simulink model "inch"  (R2023b)
settings: Solver=FixedStepAuto  StartTime=0.0  StopTime=30  RelTol=1e-3
model workspace: external: MAT-File C:\Users\Master\Desktop\seoultech_MRL\Impedance_inchworm\model_analysis\inch.mat (data not in the file)
values from neighbouring files (symbols this model uses):
  admit_d_x = 1    [inch.m]
  admit_d_z = 1    [inch.m]
  admit_k_x = 1    [inch.m]
  admit_k_z = 1    [inch.m]
  admit_m_x = 1    [inch.m]
  admit_m_z = 1    [inch.m]
  CoM1 = 0.13475    [inch.m]
  CoM2 = 0.0562    [inch.m]
  g = 9.80665    [inch.m]
  K_sp1 = 11.8    [inch.m]
  K_sp2 = 5.7    [inch.m]
  L1 = 0.24215    [inch.m]
  L2 = 0.1759    [inch.m]
  m1 = 0.420    (= 0.42)    [inch.m]
  m2 = 0.225    [inch.m]
  w_c = 30    [inch.m]
settings Model: Creator=seosu  LastModifiedBy=Master
settings RTWCC: GPUComputeCapability=5.0

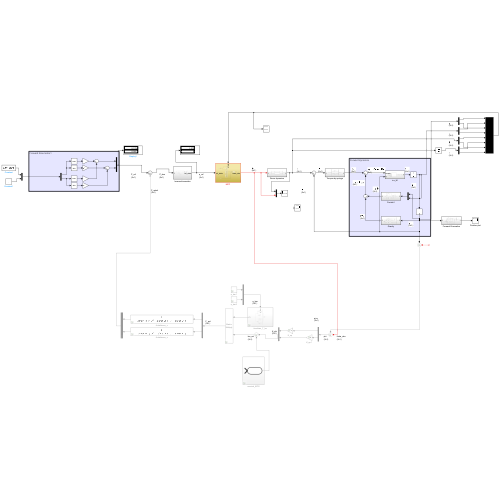
[thumbnail: Simulink's stored preview of the top-level diagram]
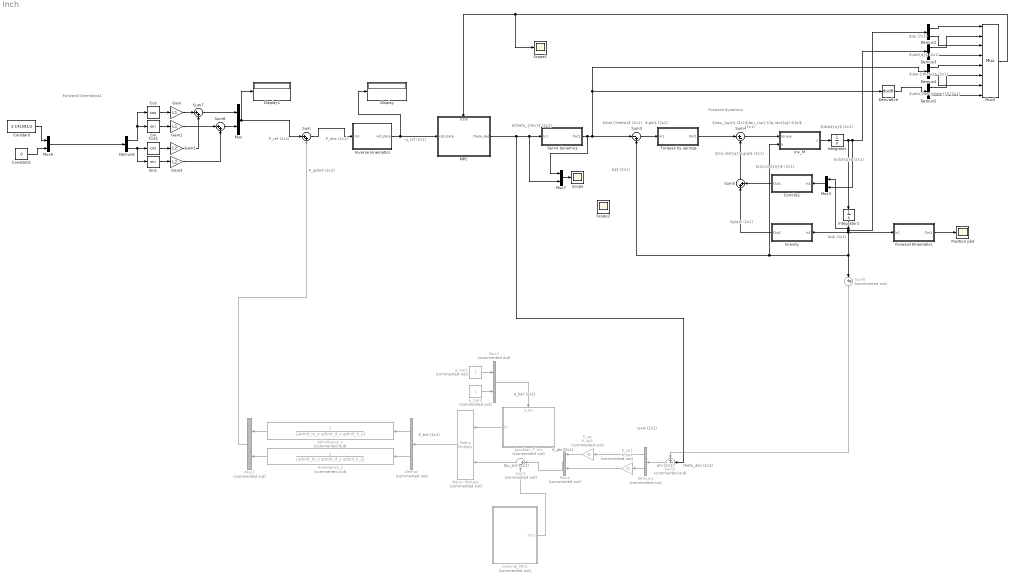
== system inch ==
  note: Forward Kinematics1
  note: P_ref
      | (2x1)
  note: q+w
      | (2x1)
  note: theta_des
      | (2x1)
  note: phi
      | (2x1)
  note: K_phi
      | (2x1)
  note: tau_ext
      | (2x1)
  note: F_ext
      | (2x1)
  note: q_bar
      | (2x1)
  note: P_admit
      | (2x1)
  note: P_des
      | (2x1)
  note: Forward dynamics
  note: q_ref
      | (2x1)
  note: $\theta_{des}$
      | (2x1)
  note: $\bar{\theta}$
      | (2x1)
  note: $q$
      | (2x1)
  note: $\phi$
      | (2x1)
  note: $\tau_{sp}$
      | (2x1)
  note: $\tau_{sp}-C(q,\dot{q})-G(q)$
      | (2x1)
  note: $g(q)$
      | (2x1)
  note: $c(q,\dot{q})$
      | (2x1)
  note: $c(q,\dot{q})+g(q)$
      | (2x1)
  note: $\ddot{q}$
      | (2x1)
  note: $\dot{q}$
      | (2x1)
  note: $q$
      | (2x1)
  note: $q$
      | (2x1)
  note: $\dot{q}$
      | (2x1)
  note: $\bar{\theta}$
      | (2x1)
  note: $\dot{\bar{\theta}}$
      | (2x1)
  Admittance_x : TransferFcn  Commented=on  Denominator=[admit_m_x admit_d_x admit_k_x]
  Admittance_z : TransferFcn  Commented=on  Denominator=[admit_m_z admit_d_z admit_k_z]
  Constant : Constant  Value=3.141592/2
  Constant1 : Constant  Value=0
  Coriolis1 : Subsystem
  Cos : Trigonometry  Operator=cos
  Cos1 : Trigonometry  Operator=cos
  Demux : Demux  Commented=on  Outputs=2
  Demux1 : Demux  Commented=on  Outputs=2
  Demux{2..6} (5 alike) : Demux  Outputs=2
  Derivative : Derivative
  Display : Display
  Display1 : Display
  Forward Kinematics : Subsystem
  Gain : Gain  Gain=L1
  Gain1 : Gain  Gain=L1
  Gain2 : Gain  Gain=L2
  Gain3 : Gain  Gain=L2
  Gravity : Subsystem
  Integrator : Integrator
  Integrator1 : Integrator
  Inverse kinematics : Subsystem
  Jacobian_T_Inv : Subsystem  Commented=on
      settings: PortSchema="{\"entries\":[{\"content\":{\"sides\":[{\"content\":{},\"type\":\"ConnectorPlacement.EquallySpacedRectSide\",\"uuid\":\"e35815a1-46bf-4be5-848e-f0ce23dcfc5f\"},{\"content\":{\"connectorIds\":[\"Out1\"],\"side\":\"RIGHT\"},\"type\":\"ConnectorPlacement.EquallySpacedRectSide\",\"uuid\":\"475e0ecd-9b25-4f4d-9a47-e60ebdf6c1c0\"},{\"content\":{\"connectorIds\":[\"In1\"],\"side\":\"TOP\"},\"type\":\"ConnectorPlacement.EquallySpacedRectSide\",\"uuid\":\"24b4edd2-9023-4e45-b53e-92ef1b268f51\"}]},\"type\":\"ConnectorPlacement.EquallySpacedConnector\",\"uuid\":\"0e42b979-70d4-4e07-81ad-a6fcf3fd88d3\"}],\"packageUris\":[\"http://schema.mathworks.com/mf0/Connector/R2020b\"],\"version\":\"1.0\"}"
  K_sp : Gain  Commented=on  Gain=K_sp1
  K_sp1 : Gain  Commented=on  Gain=K_sp2
  MPC : Subsystem
      settings: PortSchema="{\"entries\":[{\"content\":{\"sides\":[{\"content\":{\"connectorIds\":[\"In1\"]},\"type\":\"ConnectorPlacement.EquallySpacedRectSide\",\"uuid\":\"faaa2caa-5b70-4c85-ac0e-3ca1c201351b\"},{\"content\":{\"connectorIds\":[\"Out1\"],\"side\":\"RIGHT\"},\"type\":\"ConnectorPlacement.EquallySpacedRectSide\",\"uuid\":\"30f98641-3e3d-4ab7-bed4-d131e440aef7\"},{\"content\":{\"connectorIds\":[\"In2\"],\"side\":\"TOP\"},\"type\":\"ConnectorPlacement.EquallySpacedRectSide\",\"uuid\":\"cc9bccd0-31f7-44f6-a189-fb05f25d7f1a\"}]},\"type\":\"ConnectorPlacement.EquallySpacedConnector\",\"uuid\":\"92c981b0-7f9b-49a2-b6f3-a82ac2dd5f41\"}],\"packageUris\":[\"http://schema.mathworks.com/mf0/Connector/R2020b\"],\"version\":\"1.0\"}"
  Matrix Multiply : Product  Commented=on  Multiplication=Matrix(*)
  Mux{,3,6..7} (4 alike) : Mux  Inputs=2
  Mux1 : Mux  Commented=on  Inputs=2
  Mux2 : Mux  Commented=on  Inputs=2
  Mux4 : Mux  Commented=on  Inputs=2
  Mux5 : Mux  Inputs=8
  Position plot : Scope
  Scope : Scope
  Scope1 : Scope
  Scope2 : Scope
  Servo dynamics : Subsystem
  Sin : Trigonometry
  Sin1 : Trigonometry
  Sum{,5,7..8} (4 alike) : Sum  Inputs=|++
  Sum1 : Sum  Commented=on  Inputs=|+-
  Sum2 : Sum  Commented=on  Inputs=+-|
  Sum3 : Sum  Inputs=|-+
  Sum4 : Sum  Inputs=|+-
  Sum6 : Sum  Commented=on  Inputs=|++
  Torques by springs : Subsystem
  inv_M : Subsystem
  nominal_MCG : Subsystem  Commented=on
  q_bar1 : Constant  Commented=on  Value=2
  q_bar2 : Constant  Commented=on
  wires:
  Mux/1 -> Sum/1, Display1/1
  Mux2/1 -> Jacobian_T_Inv/1(q_bar)
  Jacobian_T_Inv/1(JTI) -> Matrix Multiply/1
  Matrix Multiply/1 -> Demux/1
  Sum1/1 -> Matrix Multiply/2
  nominal_MCG/1(Out1) -> Sum1/2
  Sum2/1 -> Demux1/1
  Integrator1/1 -> inv_M/2(q), Sum3/2, Sum6/1, Gravity/1(In1), Forward Kinematics/1(In1), Demux2/1, Mux3/1
  Admittance_x/1 -> Mux1/1
  Demux/2 -> Admittance_z/1
  Admittance_z/1 -> Mux1/2
  Demux/1 -> Admittance_x/1
  q_bar1/1 -> Mux2/1
  q_bar2/1 -> Mux2/2
  MPC/1(theta_des) -> Mux7/2, Servo dynamics/1(In1), Sum2/2
  Torques by springs/1(Out1) -> Sum4/1
  Sum4/1 -> inv_M/1(torque)
  Sum3/1 -> Torques by springs/1(In1)
  Derivative/1 -> Demux5/1
  inv_M/1(y) -> Integrator/1
  Integrator/1 -> Demux3/1, Mux3/2, Integrator1/1
  Forward Kinematics/1(Out1) -> Position plot/1
  Sum5/1 -> Sum4/2
  Servo dynamics/1(Out1) -> Mux7/1, Demux4/1, Derivative/1, Sum3/1
  Gravity/1(Out1) -> Sum5/1
  Coriolis1/1(Out1) -> Sum5/2
  Sum6/1 -> Sum2/1
  ? -> Sum6/2
  Mux3/1 -> Coriolis1/1(In1)
  Demux1/1 -> K_sp/1
  Demux1/2 -> K_sp1/1
  K_sp1/1 -> Mux4/2
  K_sp/1 -> Mux4/1
  Mux4/1 -> Sum1/1
  Inverse kinematics/1(ref_state) -> Display/1, MPC/1(ref_state)
  Sum/1 -> Inverse kinematics/1(In1)
  Demux2/1 -> Mux5/1
  Demux2/2 -> Mux5/3
  Demux3/1 -> Mux5/2
  Demux3/2 -> Mux5/4
  Demux4/1 -> Mux5/5
  Demux5/1 -> Mux5/6
  Demux4/2 -> Mux5/7
  Demux5/2 -> Mux5/8
  Mux5/1 -> Scope1/1, MPC/2(state)
  Sum8/1 -> Mux/2
  Sum7/1 -> Mux/1
  Gain3/1 -> Sum8/2
  Gain1/1 -> Sum8/1
  Gain/1 -> Sum7/1
  Gain2/1 -> Sum7/2
  Sin/1 -> Gain1/1
  Sin1/1 -> Gain3/1
  Cos1/1 -> Gain2/1
  Cos/1 -> Gain/1
  Demux6/2 -> Sin1/1, Cos1/1
  Demux6/1 -> Cos/1, Sin/1
  Mux6/1 -> Demux6/1
  Constant/1 -> Mux6/1
  Constant1/1 -> Mux6/2
  Mux7/1 -> Scope/1
  Mux1/1 -> Sum/2

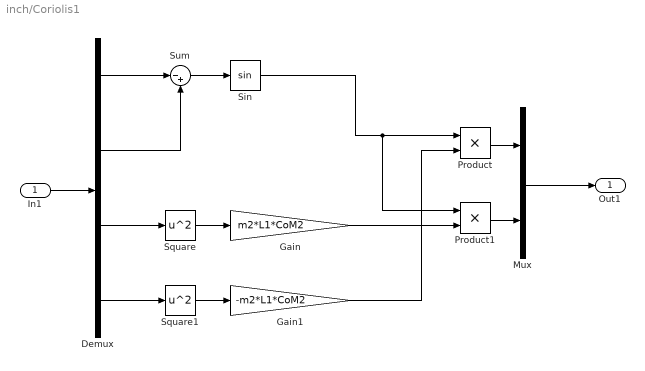
== system inch/Coriolis1 ==
  In1 : Inport
  Demux : Demux
  Gain : Gain  Gain=m2*L1*CoM2
  Gain1 : Gain  Gain=-m2*L1*CoM2
  Mux : Mux  Inputs=2
  Product : Product
  Product1 : Product
  Sin : Trigonometry
  Square : Math  Operator=square  SignedPower=on  RndMeth=Zero
  Square1 : Math  Operator=square  SignedPower=on  RndMeth=Zero
  Sum : Sum  Inputs=|-+
  Out1 : Outport
  wires:
  In1/1 -> Demux/1
  Demux/2 -> Sum/2
  Demux/1 -> Sum/1
  Sum/1 -> Sin/1
  Demux/3 -> Square/1
  Demux/4 -> Square1/1
  Square/1 -> Gain/1
  Square1/1 -> Gain1/1
  Sin/1 -> Product1/1, Product/1
  Gain/1 -> Product1/2
  Gain1/1 -> Product/2
  Product1/1 -> Mux/2
  Product/1 -> Mux/1
  Mux/1 -> Out1/1

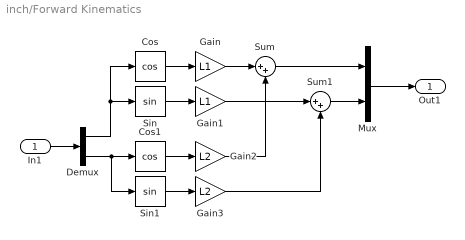
== system inch/Forward Kinematics ==
  In1 : Inport
  Cos : Trigonometry  Operator=cos
  Cos1 : Trigonometry  Operator=cos
  Demux : Demux  Outputs=2
  Gain : Gain  Gain=L1
  Gain1 : Gain  Gain=L1
  Gain2 : Gain  Gain=L2
  Gain3 : Gain  Gain=L2
  Mux : Mux  Inputs=2
  Sin : Trigonometry
  Sin1 : Trigonometry
  Sum : Sum  Inputs=|++
  Sum1 : Sum  Inputs=|++
  Out1 : Outport
  wires:
  In1/1 -> Demux/1
  Mux/1 -> Out1/1
  Demux/1 -> Cos/1, Sin/1
  Demux/2 -> Sin1/1, Cos1/1
  Cos/1 -> Gain/1
  Cos1/1 -> Gain2/1
  Sin1/1 -> Gain3/1
  Sin/1 -> Gain1/1
  Gain2/1 -> Sum/2
  Gain/1 -> Sum/1
  Gain1/1 -> Sum1/1
  Gain3/1 -> Sum1/2
  Sum/1 -> Mux/1
  Sum1/1 -> Mux/2

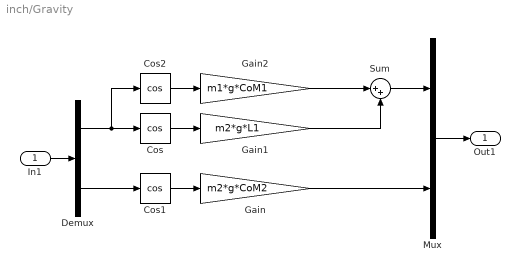
== system inch/Gravity ==
  In1 : Inport
  Cos : Trigonometry  Operator=cos
  Cos1 : Trigonometry  Operator=cos
  Cos2 : Trigonometry  Operator=cos
  Demux : Demux  Outputs=2
  Gain : Gain  Gain=m2*g*CoM2
  Gain1 : Gain  Gain=m2*g*L1
  Gain2 : Gain  Gain=m1*g*CoM1
  Mux : Mux  Inputs=2
  Sum : Sum  Inputs=|++
  Out1 : Outport
  wires:
  In1/1 -> Demux/1
  Demux/2 -> Cos1/1
  Cos1/1 -> Gain/1
  Cos2/1 -> Gain2/1
  Cos/1 -> Gain1/1
  Demux/1 -> Cos2/1, Cos/1
  Gain2/1 -> Sum/1
  Gain1/1 -> Sum/2
  Gain/1 -> Mux/2
  Sum/1 -> Mux/1
  Mux/1 -> Out1/1

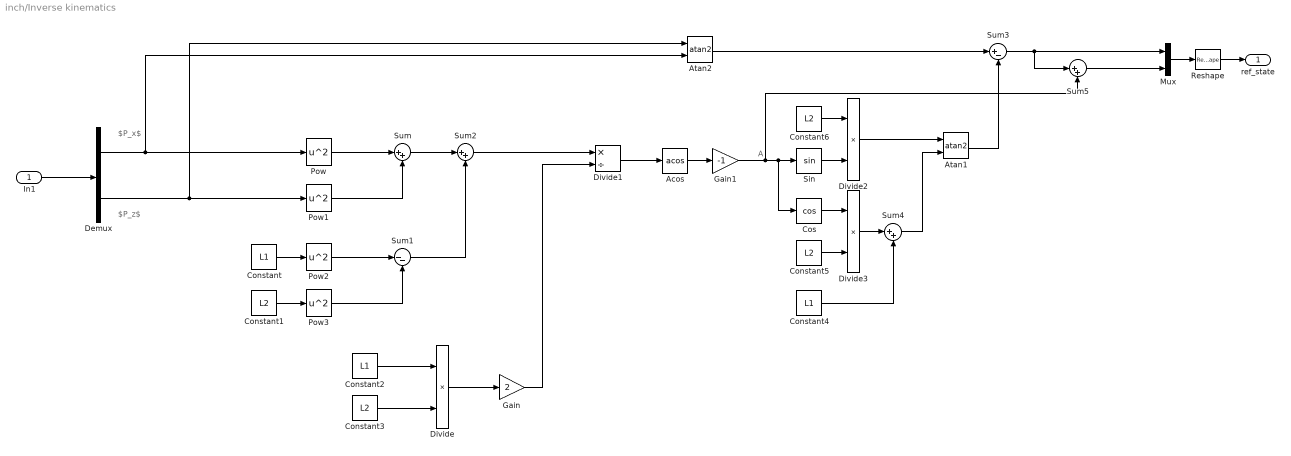
== system inch/Inverse kinematics ==
  note: A
  note: $P_x$
  note: $P_z$
  In1 : Inport
  Acos : Trigonometry  Operator=acos
  Atan1 : Trigonometry  Operator=atan2
  Atan2 : Trigonometry  Operator=atan2
  Constant : Constant  Value=L1
  Constant{1,3,5..6} (4 alike) : Constant  Value=L2
  Constant2 : Constant  Value=L1
  Constant4 : Constant  Value=L1
  Cos : Trigonometry  Operator=cos
  Demux : Demux  Outputs=2
  Divide : Product  Inputs=**
  Divide1 : Product  Inputs=*/
  Divide2 : Product  Inputs=**
  Divide3 : Product  Inputs=**
  Gain : Gain  Gain=2
  Gain1 : Gain  Gain=-1
  Mux : Mux  Inputs=2
  Pow{,1..3} (4 alike) : Math  Operator=square  SignedPower=on  RndMeth=Zero
  Reshape : Reshape  OutputDimensionality=Column vector (2-D)
  Sin : Trigonometry
  Sum{,2,4..5} (4 alike) : Sum  Inputs=|++
  Sum1 : Sum  Inputs=|--
  Sum3 : Sum  Inputs=|+-
  ref_state : Outport
  wires:
  In1/1 -> Demux/1
  Demux/1 -> Pow/1, Atan2/2
  Demux/2 -> Atan2/1, Pow1/1
  Pow/1 -> Sum/1
  Pow1/1 -> Sum/2
  Constant/1 -> Pow2/1
  Constant1/1 -> Pow3/1
  Pow2/1 -> Sum1/1
  Pow3/1 -> Sum1/2
  Sum/1 -> Sum2/1
  Sum1/1 -> Sum2/2
  Sum2/1 -> Divide1/1
  Constant2/1 -> Divide/1
  Constant3/1 -> Divide/2
  Divide/1 -> Gain/1
  Gain/1 -> Divide1/2
  Divide1/1 -> Acos/1
  Acos/1 -> Gain1/1
  Atan2/1 -> Sum3/1
  Gain1/1 -> Sum5/2, Cos/1, Sin/1
  Constant5/1 -> Divide3/2
  Cos/1 -> Divide3/1
  Divide3/1 -> Sum4/1
  Constant4/1 -> Sum4/2
  Sin/1 -> Divide2/2
  Constant6/1 -> Divide2/1
  Sum4/1 -> Atan1/2
  Divide2/1 -> Atan1/1
  Atan1/1 -> Sum3/2
  Sum3/1 -> Sum5/1, Mux/1
  Sum5/1 -> Mux/2
  Mux/1 -> Reshape/1
  Reshape/1 -> ref_state/1

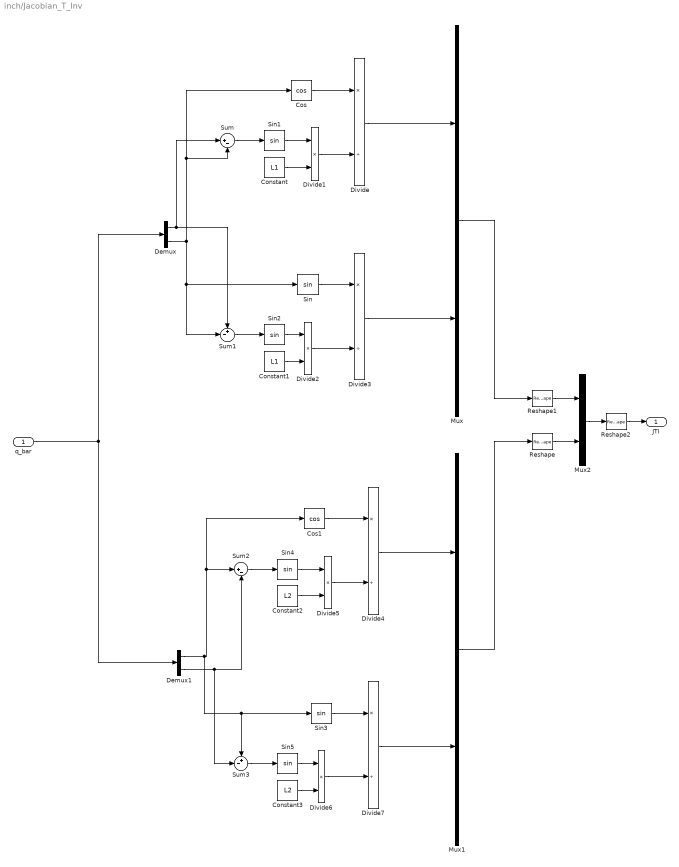
== system inch/Jacobian_T_Inv ==
  q_bar : Inport
  Constant : Constant  Value=L1
  Constant1 : Constant  Value=L1
  Constant2 : Constant  Value=L2
  Constant3 : Constant  Value=L2
  Cos : Trigonometry  Operator=cos
  Cos1 : Trigonometry  Operator=cos
  Demux : Demux  Outputs=2
  Demux1 : Demux  Outputs=2
  Divide{,3..4,7} (4 alike) : Product  Inputs=*/
  Divide{1..2,5..6} (4 alike) : Product  Inputs=**
  Mux : Mux  Inputs=2
  Mux1 : Mux  Inputs=2
  Mux2 : Mux  Inputs=2
  Reshape : Reshape  OutputDimensionality=Column vector (2-D)
  Reshape1 : Reshape  OutputDimensionality=Column vector (2-D)
  Reshape2 : Reshape  OutputDimensionality=Customize  OutputDimensions=[2,2]
  Sin{,1..5} (6 alike) : Trigonometry
  Sum : Sum  Inputs=|+-
  Sum1 : Sum  Inputs=+-|
  Sum2 : Sum  Inputs=|+-
  Sum3 : Sum  Inputs=+-|
  JTI : Outport
  wires:
  q_bar/1 -> Demux1/1, Demux/1
  Demux/2 -> Sum1/2, Sin/1, Sum/2, Cos/1
  Cos/1 -> Divide/1
  Demux/1 -> Sum/1, Sum1/1
  Sum/1 -> Sin1/1
  Sin1/1 -> Divide1/1
  Constant/1 -> Divide1/2
  Divide1/1 -> Divide/2
  Sum1/1 -> Sin2/1
  Constant1/1 -> Divide2/2
  Sin2/1 -> Divide2/1
  Divide2/1 -> Divide3/2
  Sin/1 -> Divide3/1
  Divide3/1 -> Mux/2
  Divide/1 -> Mux/1
  Divide7/1 -> Mux1/2
  Sin5/1 -> Divide6/1
  Sum3/1 -> Sin5/1
  Constant3/1 -> Divide6/2
  Divide4/1 -> Mux1/1
  Sin3/1 -> Divide7/1
  Divide6/1 -> Divide7/2
  Divide5/1 -> Divide4/2
  Sin4/1 -> Divide5/1
  Demux1/1 -> Sin3/1, Sum3/1, Cos1/1, Sum2/1
  Cos1/1 -> Divide4/1
  Constant2/1 -> Divide5/2
  Sum2/1 -> Sin4/1
  Demux1/2 -> Sum3/2, Sum2/2
  Mux/1 -> Reshape1/1
  Mux1/1 -> Reshape/1
  Mux2/1 -> Reshape2/1
  Reshape1/1 -> Mux2/1
  Reshape/1 -> Mux2/2
  Reshape2/1 -> JTI/1

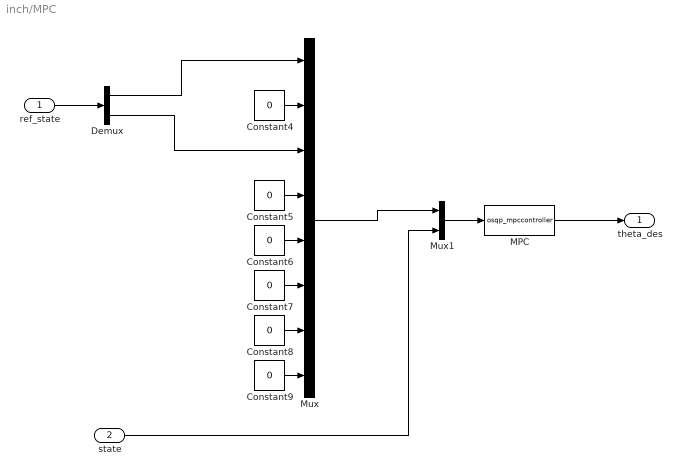
== system inch/MPC ==
  ref_state : Inport
  state : Inport  Port=2
  Constant{4..9} (6 alike) : Constant  Value=0
  Demux : Demux  Outputs=2
  MPC : MATLABFcn  MATLABFcn=osqp_mpccontroller  OutputDimensions=2  OutputSignalType=real  Output1D=off
  Mux : Mux  Inputs=8
  Mux1 : Mux  Inputs=2
  theta_des : Outport
  wires:
  ref_state/1 -> Demux/1
  Demux/1 -> Mux/1
  Demux/2 -> Mux/3
  Constant4/1 -> Mux/2
  Constant5/1 -> Mux/4
  Constant6/1 -> Mux/5
  Constant9/1 -> Mux/8
  Constant8/1 -> Mux/7
  Constant7/1 -> Mux/6
  Mux1/1 -> MPC/1
  Mux/1 -> Mux1/1
  MPC/1 -> theta_des/1
  state/1 -> Mux1/2

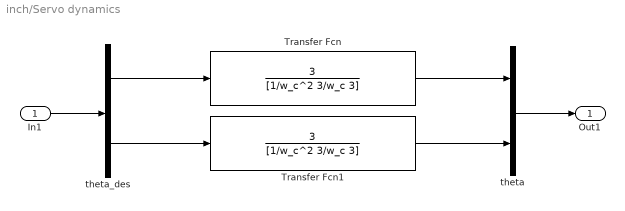
== system inch/Servo dynamics ==
  In1 : Inport
  Transfer Fcn : TransferFcn  Numerator=[3]  Denominator=[1/w_c^2 3/w_c 3]
  Transfer Fcn1 : TransferFcn  Numerator=[3]  Denominator=[1/w_c^2 3/w_c 3]
  theta : Mux  Inputs=2
  theta_des : Demux  Outputs=2
  Out1 : Outport
  wires:
  In1/1 -> theta_des/1
  theta_des/1 -> Transfer Fcn/1
  theta_des/2 -> Transfer Fcn1/1
  theta/1 -> Out1/1
  Transfer Fcn/1 -> theta/1
  Transfer Fcn1/1 -> theta/2

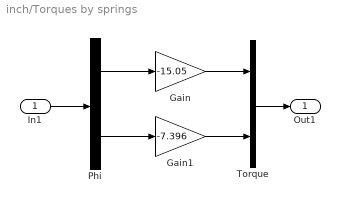
== system inch/Torques by springs ==
  In1 : Inport
  Gain : Gain  Gain=-15.05
  Gain1 : Gain  Gain=-7.396
  Phi : Demux  Outputs=2
  Torque : Mux  Inputs=2
  Out1 : Outport
  wires:
  In1/1 -> Phi/1
  Torque/1 -> Out1/1
  Gain/1 -> Torque/1
  Gain1/1 -> Torque/2
  Phi/1 -> Gain/1
  Phi/2 -> Gain1/1

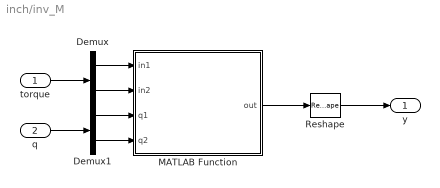
== system inch/inv_M ==
  torque : Inport
  q : Inport  Port=2
  Demux : Demux  Outputs=2
  Demux1 : Demux  Outputs=2
  MATLAB Function : MATLAB Function  TreatAsAtomicUnit=on
  Reshape : Reshape  OutputDimensionality=Column vector (2-D)
  y : Outport
  wires:
  MATLAB Function/1(out) -> Reshape/1
  torque/1 -> Demux/1
  Demux/1 -> MATLAB Function/1(in1)
  Reshape/1 -> y/1
  q/1 -> Demux1/1
  Demux/2 -> MATLAB Function/2(in2)
  Demux1/1 -> MATLAB Function/3(q1)
  Demux1/2 -> MATLAB Function/4(q2)

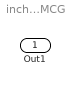
== system inch/nominal_MCG ==
  Out1 : Outport

== matlab function inch/inv_M/MATLAB Function ==
  data: in1 input; out output; in2 input; q1 input; q2 input
function out = fcn(in1, in2, q1, q2)
    L1 = 0.24215;
    L2 = 0.1759;  
    CoM1 = 0.13475;
    CoM2 = 0.0562;
    m1 = 0.420;     
    m2 = 0.225;  
    J1 = m1*L1^2/12 + m1*(CoM1-L1/2)^2;  
    J2 = m2*L2^2/12 + m2*(L2/2-CoM2)^2; 

    M = [ m1*CoM1^2+J1+m2*L1^2, m2*L1*CoM2*cos(q2-q1);
         m2*L1*CoM2*cos(q2-q1),          m2*CoM2^2+J2];
    
    
    [U, S, V] = svd(M);
    N = V * diag(1./diag(S)) * U';
    N=M;
    
    out1 = N(1,1)*in1 + N(1,2)*in2;
    out2 = N(2,1)*in1 + N(2,2)*in2;
    
    out = [out1, out2]';

end
